simulink model "controller_estimator_test"  (R2016b)
settings: Solver=VariableStepAuto  StartTime=0.0  StopTime=10.0  RelTol=1e-3
undefined symbols (not defined in the file or in its folder): fsw_params, GPS, mag_body_T, measurements_deg_err, omega_radps_gyro, sun_body_unit_photodiode, sun_body_unit_sunsensor
libraries: dynamics_lib x3, aerolibutil x2, extended_kalman_filter_lib x1, gps x1, GPS_time_lib x1, momentum_dump_lib x1, pd_control_lib x1, RW_assembly_simple_lib x1, bus_stubs_template x1, disturbances_lib x1, MSP_FSW_lib x1, gyroscope_lib x1
settings Model: Creator=sexymathemagician  LastModifiedBy=taylorreynolds

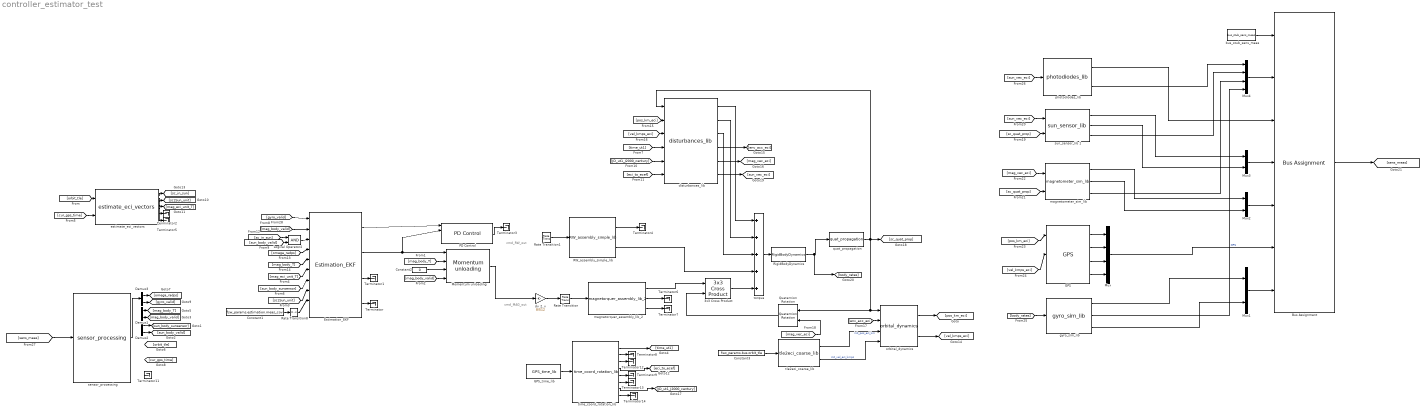
== system controller_estimator_test ==
  note: cmd_RW_out
  note: cmd_MAG_out
  3x3 Cross Product : aerolibutil/3x3 Cross Product
  Bus Assignment : BusAssignment  AssignedSignals=measurements_deg_err,sun_body_unit_photodiode,sun_body_unit_sunsensor,mag_body_T,GPS,omega_radps_gyro
  Constant1 : Constant  Value=fsw_params.estimation.meas_cov
  Constant2 : Constant  Value=0
  Constant3 : Constant  Value=fsw_params.bus.orbit_tle
  Demux1 : Demux  Outputs=[3 1]
  Demux2 : Demux  Outputs=[3 1]
  Demux3 : Demux  Outputs=[3 1]
  "Estimation_EKF " : extended_kalman_filter_lib/Estimation_EKF 
  GPS : gps/GPS
  GPS_time_lib : GPS_time_lib/GPS_time_lib
  Logical Operator2 : Logic  AllPortsSameDT=off  OutDataTypeStr=boolean
  Momentum unloading : momentum_dump_lib/Momentum unloading
  Mux : Mux  Inputs=[3 3 2 1]
  Mux1 : Mux  Inputs=[3 1]
  Mux2 : Mux  Inputs=[3 1]
  Mux3 : Mux  Inputs=[3 1]
  Mux4 : Mux
  PD Control : pd_control_lib/PD Control
  Quaternion Rotation : aerolibutil/Quaternion Rotation
  RW_assembly_simple_lib : RW_assembly_simple_lib/RW_assembly_simple_lib  natural_frequency=sim_params.actuators.reaction_wheel.natural_freq  damping_ratio=sim_params.actuators.reaction_wheel.damping  max_rate=sim_params.actuators.reaction_wheel.rate_limit
  Rate Transition : RateTransition  OutPortSampleTime=1/20
  Rate Transition1 : RateTransition  OutPortSampleTime=1/20
  Rate Transition8 : RateTransition  OutPortSampleTime=fsw_params.sample_time_s
  RigidBodyDynamics : dynamics_lib/Dynamics/RigidBodyDynamics
  Terminator{,1..9,11..14} (14 alike) : Terminator
  bus_stub_sens_meas : bus_stubs_template/bus_stub_sens_meas
  disturbances_lib : disturbances_lib/disturbances_lib
  dv_2_v : Gain  Gain=8/512
  estimate_eci_vectors : MSP_FSW_lib/MSP_FSW/estimate_eci_vectors
  gyro_sim_lib : gyroscope_lib/gyro_sim_lib
  magnetometer_sim_lib : magnetometer_lib/magnetometer_sim_lib
  magnetorquer_assembly_lib_2 : actuators_lib/Actuators/magnetorquer_assembly_lib_2
  orbital_dynamics : dynamics_lib/Dynamics/orbital_dynamics
  photodiodes_lib : photodiodes_lib/photodiodes_lib
  quat_propagation : dynamics_lib/Dynamics/quat_propagation
  sensor_processing : sensor_processing/sensor_processing
  sun_sensor_lib 1 : sun_sensor_lib/sun_sensor_lib 
  time_coord_rotation_lib : time_coord_rotation_lib/time_coord_rotation_lib
  tle2eci_coarse_lib : tle2eci_coarse_lib/tle2eci_coarse_lib
  torque : Sum  Inputs=5
  wires:
  [mag_eci_unit_T] -> "Estimation_EKF "/6
  [sc2sun_unit] -> "Estimation_EKF "/8
  [sun_body_sunsensor] -> "Estimation_EKF "/7
  "Estimation_EKF "/3 -> Terminator1/1
  "Estimation_EKF "/4 -> Terminator/1
  [mag_body_T] -> "Estimation_EKF "/5
  [omega_radps] -> "Estimation_EKF "/4
  [sc_in_sun] -> Logical Operator2/1
  [sun_body_valid] -> Logical Operator2/2
  Logical Operator2/1 -> "Estimation_EKF "/3
  [gyro_valid] -> "Estimation_EKF "/1
  [mag_body_valid] -> "Estimation_EKF "/2
  Rate Transition8/1 -> "Estimation_EKF "/9
  Constant1/1 -> Rate Transition8/1
  estimate_eci_vectors/5 -> Terminator5/1
  estimate_eci_vectors/4 -> Terminator2/1
  estimate_eci_vectors/3 -> [mag_eci_unit_T]
  estimate_eci_vectors/2 -> [sc2sun_unit]
  estimate_eci_vectors/1 -> [sc_in_sun]
  Constant2/1 -> Momentum unloading/3
  Momentum unloading/1 -> dv_2_v/1
  ? -> Rate Transition1/1
  PD Control/1 -> Terminator3/1
  [mag_body_T] -> Momentum unloading/2
  "Estimation_EKF "/2 -> PD Control/2, Momentum unloading/1
  "Estimation_EKF "/1 -> PD Control/1
  [mag_body_valid] -> Momentum unloading/4
  ? -> [orbit_tle]
  ? -> Terminator11/1
  ? -> [cur_gps_time]
  ? -> Demux2/1
  ? -> Demux1/1
  [orbit_tle] -> estimate_eci_vectors/1
  [cur_gps_time] -> estimate_eci_vectors/2
  Demux1/1 -> [mag_body_T]
  Demux1/2 -> [mag_body_valid]
  Demux2/1 -> [sun_body_sunsensor]
  Demux2/2 -> [sun_body_valid]
  Rate Transition1/1 -> RW_assembly_simple_lib/1
  dv_2_v/1 -> Rate Transition/1
  Rate Transition/1 -> magnetorquer_assembly_lib_2/1
  RW_assembly_simple_lib/1 -> Terminator4/1
  magnetorquer_assembly_lib_2/2 -> Terminator6/1
  magnetorquer_assembly_lib_2/3 -> Terminator7/1
  torque/1 -> RigidBodyDynamics/1
  disturbances_lib/3 -> torque/3
  disturbances_lib/2 -> torque/2
  disturbances_lib/1 -> torque/1
  RW_assembly_simple_lib/2 -> torque/4
  RigidBodyDynamics/1 -> [body_rates], quat_propagation/1
  quat_propagation/1 -> [sc_quat_prop], Quaternion Rotation/1, orbital_dynamics/1, disturbances_lib/1
  magnetorquer_assembly_lib_2/1 -> 3x3 Cross Product/1
  Quaternion Rotation/1 -> 3x3 Cross Product/2
  3x3 Cross Product/1 -> torque/5
  GPS_time_lib/1 -> time_coord_rotation_lib/1
  time_coord_rotation_lib/4 -> [eci_to_ecef]
  time_coord_rotation_lib/7 -> [JD_ut1_J2000_century]
  time_coord_rotation_lib/2 -> Terminator8/1
  time_coord_rotation_lib/1 -> [time_ut1]
  time_coord_rotation_lib/5 -> Terminator9/1
  [eci_to_ecef] -> disturbances_lib/6
  [JD_ut1_J2000_century] -> disturbances_lib/5
  [time_ut1] -> disturbances_lib/4
  [pos_km_eci] -> disturbances_lib/2
  orbital_dynamics/1 -> [pos_km_eci]
  orbital_dynamics/2 -> [vel_kmps_eci]
  [vel_kmps_eci] -> disturbances_lib/3
  disturbances_lib/4 -> [env_acc_eci]
  [env_acc_eci] -> orbital_dynamics/2
  Constant3/1 -> tle2eci_coarse_lib/1
  tle2eci_coarse_lib/1 -> orbital_dynamics/3  "init_pos_eci_km"
  tle2eci_coarse_lib/2 -> orbital_dynamics/4  "init_vel_eci_kmps"
  disturbances_lib/5 -> [mag_vec_eci]
  [mag_vec_eci] -> Quaternion Rotation/2
  [sc_quat_prop] -> sun_sensor_lib 1/2
  disturbances_lib/6 -> [sun_vec_eci]
  [sun_vec_eci] -> sun_sensor_lib 1/1
  [sc_quat_prop] -> magnetometer_sim_lib/2
  [mag_vec_eci] -> magnetometer_sim_lib/1
  [pos_km_eci] -> GPS/1
  [vel_kmps_eci] -> GPS/2
  [body_rates] -> gyro_sim_lib/1
  bus_stub_sens_meas/1 -> Bus Assignment/1
  [sun_vec_eci] -> photodiodes_lib/1
  Mux4/1 -> Bus Assignment/2
  photodiodes_lib/1 -> Bus Assignment/3
  photodiodes_lib/2 -> Mux4/1
  Mux3/1 -> Bus Assignment/4
  sun_sensor_lib 1/1 -> Mux3/1
  sun_sensor_lib 1/2 -> Mux3/2
  sun_sensor_lib 1/3 -> Mux4/2
  Mux2/1 -> Bus Assignment/5
  magnetometer_sim_lib/1 -> Mux2/1
  magnetometer_sim_lib/2 -> Mux2/2
  magnetometer_sim_lib/3 -> Mux4/3
  GPS/4 -> Mux/4
  Mux/1 -> Bus Assignment/6  "GPS"
  GPS/3 -> Mux/3
  GPS/2 -> Mux/2
  GPS/1 -> Mux/1
  gyro_sim_lib/2 -> Mux4/4
  Mux1/1 -> Bus Assignment/7
  gyro_sim_lib/1 -> Mux1/1
  gyro_sim_lib/3 -> Mux1/2
  Bus Assignment/1 -> [sens_meas]
  [sens_meas] -> sensor_processing/1
  sensor_processing/1 -> Demux3/1
  Demux3/1 -> [omega_radps]
  Demux3/2 -> [gyro_valid]
  time_coord_rotation_lib/3 -> Terminator12/1
  time_coord_rotation_lib/6 -> Terminator13/1
  time_coord_rotation_lib/8 -> Terminator14/1
